simulink model "torqueWalkingR2012b"  (Simulink 8.0)
settings: Solver=FixedStepDiscrete  StartTime=0.0  StopTime=Config.t_end  FixedStep=Config.t_step  RelTol=1e-3
InitFcn:
  | cd(fileparts(which(bdroot)));
  | initTorqueWalking;
StopFcn:
  | disp_early_termination
undefined symbols (not defined in the file or in its folder): biasVectorConstraint_feet, Config, ConstraintMatrix_feet, DiscIntNeverNeededParam, Gains, ROBOT_DOF, Sat
libraries: WBToolboxLibrary x114, simulink x2
(part 2 of 4)

== system torqueWalkingR2012b/Robot State and References/State Machines ==
  Compute Feet to Base Link Transforms : Subsystem
  Compute State Velocity : Subsystem
  Constant6 : Constant  Value=eye(4)
  Get Estimate : WBToolboxLibrary/wholeBodyStates/Get Estimate  estimateType=Joints Position  robotName=WBT_robotName  localName=WBT_modelName  wbiFile=WBT_wbiFilename  wbiList=WBT_wbiList
  Get Estimate1 : WBToolboxLibrary/wholeBodyStates/Get Estimate  estimateType=Joints Velocity  robotName=WBT_robotName  localName=WBT_modelName  wbiFile=WBT_wbiFilename  wbiList=WBT_wbiList
  IMU measurements : WBToolboxLibrary/Utilities/Yarp Read  portName=Ports.IMU  signalSize=12  blocking=off  timestamp=off  autoconnect=on  errorOnConnection=off
  Select the Current State and References : Subsystem
  Selector1 : Selector  NumberOfDimensions=2  InputPortWidth=ROBOT_DOF  IndexOptions=Index vector (dialog),Index vector (dialog)  Indices=[1:ROBOT_DOF],1  OutputSizes=1,1
  s : Outport
  w_H_b : Outport  Port=2
  nu : Outport  Port=3
  feetInContact : Outport  Port=4
  state : Outport  Port=5
  references_LFoot : Outport  Port=6
  references_RFoot : Outport  Port=7
  references_CoM : Outport  Port=8
  references_rot_task : Outport  Port=9
  references_LHand : Outport  Port=10
  references_RHand : Outport  Port=11
  references_s : Outport  Port=12
  tag scope: feetInContact=global, nu=global, s=global, s_des=global, sd=global, state=global, w_H_b=global
  wires:
  Get Estimate/1 -> Compute State Velocity/2(s), s/1, [s], Select the Current State and References/1(s), Compute Feet to Base Link Transforms/1(s)
  Constant6/1 -> Compute Feet to Base Link Transforms/2(w_H_base_fixed)
  IMU measurements/1 -> Compute Feet to Base Link Transforms/3(IMU port)
  Compute Feet to Base Link Transforms/1(fixed_link_H_b) -> Select the Current State and References/2(fixed_link_H_b)
  Select the Current State and References/1(w_H_b) -> w_H_b/1, [w_H_b], Compute State Velocity/3(w_H_b)
  Select the Current State and References/2(feetInContact) -> feetInContact/1, [feetInContact], Compute State Velocity/4("feetInContact ")
  Compute State Velocity/1(nu) -> nu/1, [nu]
  Select the Current State and References/3(state) -> [state], state/1
  Select the Current State and References/10(references_s) -> references_s/1, Selector1/1
  Select the Current State and References/6(references_CoM) -> references_CoM/1
  Select the Current State and References/7(references_rot_task) -> references_rot_task/1
  Select the Current State and References/5(references_RFoot) -> references_RFoot/1
  Select the Current State and References/4(references_LFoot) -> references_LFoot/1
  Selector1/1 -> [s_des]
  Compute Feet to Base Link Transforms/2(LFoot_H_b) -> Select the Current State and References/3(LFoot_H_b)
  Compute Feet to Base Link Transforms/3(RFoot_H_b) -> Select the Current State and References/4(RFoot_H_b)
  Select the Current State and References/8(references_LHand) -> references_LHand/1
  Select the Current State and References/9(references_RHand) -> references_RHand/1
  Get Estimate1/1 -> [sd], Compute State Velocity/1(Joints velocity)

== system torqueWalkingR2012b/Subsystem/ZMP, support polygon ==
  f_Lfoot : Inport
  f_Rfoot : Inport  Port=2
  pose_lFoot : Inport  Port=3
  orient_lFoot : Inport  Port=4
  pose_rFoot : Inport  Port=5
  orient_rFoot : Inport  Port=6
  feetInContact : Inport  Port=7
  state : Inport  Port=8
  compute ZMP : MATLAB Function  TreatAsAtomicUnit=on
      settings: PermitHierarchicalResolution=ParametersOnly
  supportPolygon : MATLAB Function  TreatAsAtomicUnit=on
      settings: PermitHierarchicalResolution=ParametersOnly
  zmp : Outport
  support_polygon : Outport  Port=2
  tag scope: ZMP=global, support_polygon=global
  wires:
  pose_lFoot/1 -> supportPolygon/1(pose_lFoot), compute ZMP/3(pose_lFoot)
  pose_rFoot/1 -> compute ZMP/5(pose_rFoot), supportPolygon/2(pose_rFoot)
  compute ZMP/1(ZMP) -> zmp/1, [ZMP]
  f_Lfoot/1 -> compute ZMP/1(f_lFoot)
  f_Rfoot/1 -> compute ZMP/2(f_rFoot)
  orient_lFoot/1 -> compute ZMP/4(orient_lFoot)
  orient_rFoot/1 -> compute ZMP/6(orient_rFoot)
  feetInContact/1 -> compute ZMP/7(feetInContact), supportPolygon/3(feet_in_contact)
  supportPolygon/1(supportPolygon) -> [support_polygon], support_polygon/1
  state/1 -> supportPolygon/4(state)

== system torqueWalkingR2012b/Subsystem/task errors ==
  pos_vel_CoM : Inport
  pos_vel_acc_CoM_des : Inport  Port=2
  orient_vel_rot_rask : Inport  Port=3
  pos_vel_acc_rot_task_des : Inport  Port=4
  pose_vel_LFoot : Inport  Port=5
  pos_vel_acc_LFoot_des : Inport  Port=6
  pose_vel_RFoot : Inport  Port=7
  pos_vel_acc_RFoot_des : Inport  Port=8
  Rotation Error Left Foot : Subsystem
  Rotation Error Left Foot1 : Subsystem
  Rotation Error Rotational Task : Subsystem
  Selector{,2..6} (6 alike) : Selector  NumberOfDimensions=2  InputPortWidth=3  IndexOptions=Index vector (dialog),Index vector (dialog)  Indices=[1:3],1  OutputSizes=1,1
  Selector12 : Selector  NumberOfDimensions=2  InputPortWidth=3  IndexOptions=Index vector (dialog),Index vector (dialog)  Indices=[1:3],[1:3]  OutputSizes=1,1
  Selector13 : Selector  NumberOfDimensions=2  InputPortWidth=3  IndexOptions=Index vector (dialog),Index vector (dialog)  Indices=[1:3],[1:3]  OutputSizes=1,1
  Selector{7..9,15} (4 alike) : Selector  NumberOfDimensions=2  InputPortWidth=3  IndexOptions=Index vector (dialog),Index vector (dialog)  Indices=[4:6],[1:3]  OutputSizes=1,1
  Sum : Sum  Inputs=+-|
  Sum2 : Sum  Inputs=+-|
  Sum3 : Sum  Inputs=+-|
  Vector Concatenate : Concatenate  NumInputs=6
  taskErrors : Outport
  wires:
  Rotation Error Left Foot/1(|1-R^T*RDes|^2) -> Vector Concatenate/4
  Sum3/1 -> Vector Concatenate/5
  Sum2/1 -> Vector Concatenate/3
  Selector6/1 -> Sum3/2
  Selector5/1 -> Sum3/1
  pose_vel_LFoot/1 -> Selector3/1, Selector7/1
  pose_vel_RFoot/1 -> Selector9/1, Selector5/1
  Selector4/1 -> Sum2/2
  Selector/1 -> Sum/1
  Rotation Error Left Foot1/1(|1-R^T*RDes|^2) -> Vector Concatenate/6
  Selector13/1 -> Rotation Error Rotational Task/1(w_R_rot_task)
  Selector12/1 -> Rotation Error Rotational Task/2(w_R_rot_task_des)
  pos_vel_acc_LFoot_des/1 -> Selector15/1, Selector4/1
  Selector15/1 -> Rotation Error Left Foot/2(w_R_RFoot_des)
  Sum/1 -> Vector Concatenate/1
  Rotation Error Rotational Task/1(|1-R^T*RDes|^2) -> Vector Concatenate/2
  Selector8/1 -> Rotation Error Left Foot1/2(w_R_RFoot_des)
  orient_vel_rot_rask/1 -> Selector13/1
  Selector2/1 -> Sum/2
  Selector9/1 -> Rotation Error Left Foot1/1(w_R_RFoot)
  Selector3/1 -> Sum2/1
  pos_vel_acc_rot_task_des/1 -> Selector12/1
  pos_vel_acc_RFoot_des/1 -> Selector8/1, Selector6/1
  pos_vel_CoM/1 -> Selector/1
  Selector7/1 -> Rotation Error Left Foot/1(w_R_RFoot)
  pos_vel_acc_CoM_des/1 -> Selector2/1
  Vector Concatenate/1 -> taskErrors/1

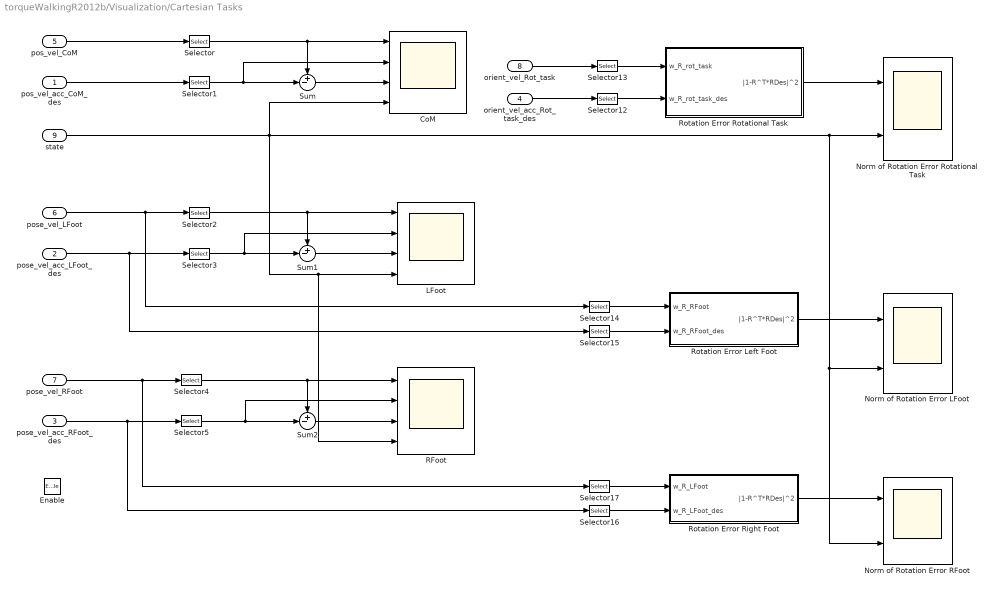
== system torqueWalkingR2012b/Visualization/Cartesian Tasks ==
  pos_vel_acc_CoM_des : Inport
  pose_vel_acc_LFoot_des : Inport  Port=2
  pose_vel_acc_RFoot_des : Inport  Port=3
  orient_vel_acc_Rot_task_des : Inport  Port=4
  pos_vel_CoM : Inport  Port=5
  pose_vel_LFoot : Inport  Port=6
  pose_vel_RFoot : Inport  Port=7
  orient_vel_Rot_task : Inport  Port=8
  state : Inport  Port=9
  Enable : EnablePort
  CoM : Scope  NumInputPorts=4
      settings: TimeRange=auto  ShowLegends=on  MaxDataPoints=5000  SaveName=forKin_CoM_DATA  YMin=-0.22134~-0.21729~-0.00986~0.5  YMax=0.60585~0.59423~0.01226~5.5  SampleTime=-1
  LFoot : Scope  NumInputPorts=4
      settings: TimeRange=auto  MaxDataPoints=5000  SaveName=forKin_LFoot_DATA  YMin=-0.0302~-0.02873~-0.00903~0.5  YMax=0.0249~0.02873~0.00291~5.5  SampleTime=-1
  Norm of Rotation Error LFoot : Scope  NumInputPorts=2
      settings: TimeRange=auto  MaxDataPoints=5000  SaveName=ScopeData2  YMin=-0.000002~0.5  YMax=0.000022~5.5  SampleTime=-1
  Norm of Rotation Error RFoot : Scope  NumInputPorts=2
      settings: TimeRange=auto  MaxDataPoints=5000  SaveName=ScopeData3  YMin=-0.00046~0.5  YMax=0.00415~5.5  SampleTime=-1
  Norm of Rotation Error Rotational Task : Scope  NumInputPorts=2
      settings: TimeRange=auto  MaxDataPoints=5000  YMin=-0.07412~0.9  YMax=0.66711~1.1  SampleTime=-1
  RFoot : Scope  NumInputPorts=4
      settings: TimeRange=auto  ShowLegends=on  MaxDataPoints=5000  SaveName=forKin_RFoot_DATA  YMin=-0.16101~-0.15882~-0.00115~0.5  YMax=0.03981~0.0433~0.00043~5.5  SampleTime=-1
  Rotation Error Left Foot : Subsystem
  Rotation Error Right Foot : Subsystem
  Rotation Error Rotational Task : Subsystem
  Selector{,1..5} (6 alike) : Selector  NumberOfDimensions=2  InputPortWidth=3  IndexOptions=Index vector (dialog),Index vector (dialog)  Indices=[1:3],1  OutputSizes=1,1
  Selector12 : Selector  NumberOfDimensions=2  InputPortWidth=3  IndexOptions=Index vector (dialog),Index vector (dialog)  Indices=[1:3],[1:3]  OutputSizes=1,1
  Selector13 : Selector  NumberOfDimensions=2  InputPortWidth=3  IndexOptions=Index vector (dialog),Index vector (dialog)  Indices=[1:3],[1:3]  OutputSizes=1,1
  Selector{14..17} (4 alike) : Selector  NumberOfDimensions=2  InputPortWidth=3  IndexOptions=Index vector (dialog),Index vector (dialog)  Indices=[4:6],[1:3]  OutputSizes=1,1
  Sum : Sum  Inputs=+-|
  Sum1 : Sum  Inputs=+-|
  Sum2 : Sum  Inputs=+-|
  wires:
  Selector1/1 -> CoM/2, Sum/2
  pos_vel_CoM/1 -> Selector/1
  pos_vel_acc_CoM_des/1 -> Selector1/1
  Selector2/1 -> Sum1/1, LFoot/1
  Selector3/1 -> Sum1/2, LFoot/2
  Selector4/1 -> Sum2/1, RFoot/1
  Selector5/1 -> RFoot/2, Sum2/2
  pose_vel_RFoot/1 -> Selector4/1, Selector17/1
  state/1 -> Norm of Rotation Error RFoot/2, Norm of Rotation Error LFoot/2, Norm of Rotation Error Rotational Task/2, CoM/4, RFoot/4, LFoot/4
  pose_vel_acc_RFoot_des/1 -> Selector5/1, Selector16/1
  pose_vel_LFoot/1 -> Selector2/1, Selector14/1
  Selector12/1 -> Rotation Error Rotational Task/2(w_R_rot_task_des)
  pose_vel_acc_LFoot_des/1 -> Selector15/1, Selector3/1
  orient_vel_acc_Rot_task_des/1 -> Selector12/1
  orient_vel_Rot_task/1 -> Selector13/1
  Selector/1 -> Sum/1, CoM/1
  Sum/1 -> CoM/3
  Sum1/1 -> LFoot/3
  Sum2/1 -> RFoot/3
  Rotation Error Rotational Task/1(|1-R^T*RDes|^2) -> Norm of Rotation Error Rotational Task/1
  Selector13/1 -> Rotation Error Rotational Task/1(w_R_rot_task)
  Rotation Error Left Foot/1(|1-R^T*RDes|^2) -> Norm of Rotation Error LFoot/1
  Selector14/1 -> Rotation Error Left Foot/1(w_R_RFoot)
  Selector15/1 -> Rotation Error Left Foot/2(w_R_RFoot_des)
  Rotation Error Right Foot/1(|1-R^T*RDes|^2) -> Norm of Rotation Error RFoot/1
  Selector16/1 -> Rotation Error Right Foot/2(w_R_LFoot_des)
  Selector17/1 -> Rotation Error Right Foot/1(w_R_LFoot)

== system torqueWalkingR2012b/Visualization/Emergency Stop ==
  note: Stop the simulation when the force on each feet is below a threshold (i.e. robot falls)
  F_l_foot : Inport
  F_r_foot : Inport  Port=2
  Enable : EnablePort
  Compare To Constant : simulink/Logic and Bit Operations/Compare To Constant  relop=<=  const=50  OutDataTypeStr=boolean
  Compare To Constant1 : simulink/Logic and Bit Operations/Compare To Constant  relop=<=  const=50  OutDataTypeStr=boolean
  Constant3 : Constant  Value=0  OutDataTypeStr=boolean
  Constant4 : Constant  OutDataTypeStr=boolean
  Logical Operator : Logic  AllPortsSameDT=off  OutDataTypeStr=boolean
  Stop Simulation : Stop
  Switch1 : Switch  Criteria=u2 ~= 0  Threshold=0.5
  To Workspace : ToWorkspace  VariableName=no_force_on_feet  SaveFormat=Timeseries  SampleTime=-1
      settings: MaxDataPoints=1
  select_pose5 : Selector  InputPortWidth=6  IndexOptions=Index vector (dialog)  Indices=[3]  OutputSizes=1
  select_pose6 : Selector  InputPortWidth=6  IndexOptions=Index vector (dialog)  Indices=[3]  OutputSizes=1
  wires:
  F_l_foot/1 -> select_pose5/1
  F_r_foot/1 -> select_pose6/1
  Compare To Constant/1 -> Logical Operator/1
  Compare To Constant1/1 -> Logical Operator/2
  Logical Operator/1 -> Switch1/2
  Switch1/1 -> To Workspace/1, Stop Simulation/1
  Constant4/1 -> Switch1/1
  Constant3/1 -> Switch1/3
  select_pose5/1 -> Compare To Constant/1
  select_pose6/1 -> Compare To Constant1/1

== system torqueWalkingR2012b/Visualization/Emergency Stop1 ==
  exitFlagQP : Inport
  Enable : EnablePort
  Constant : Constant  Value=2
  Constant1 : Constant  Value=0  OutDataTypeStr=boolean
  Constant2 : Constant  OutDataTypeStr=boolean
  Stop Simulation : Stop
  Sum : Sum  Inputs=|++
  Switch : Switch  Criteria=u2 > Threshold  Threshold=0.1
  To Workspace : ToWorkspace  VariableName=exitFlagQP_unsuccessful  SaveFormat=Timeseries  SampleTime=-1
      settings: MaxDataPoints=1
  wires:
  exitFlagQP/1 -> Sum/1
  Sum/1 -> Switch/2
  Constant/1 -> Sum/2
  Constant1/1 -> Switch/1
  Constant2/1 -> Switch/3
  Switch/1 -> To Workspace/1, Stop Simulation/1

== system torqueWalkingR2012b/Visualization/Emergency Stop2 ==
  note: Stop the simulation when the ZMP goes out of the support polygon
  ZMP : Inport
  support_polygon : Inport  Port=2
  Enable : EnablePort
  Constant3 : Constant  Value=0  OutDataTypeStr=boolean
  Constant4 : Constant  OutDataTypeStr=boolean
  Logical Operator : Logic  Operator=OR  AllPortsSameDT=off  OutDataTypeStr=boolean
  Relational Operator : RelationalOperator  Operator=<  OutDataTypeStr=boolean
  Relational Operator1 : RelationalOperator  Operator=>  OutDataTypeStr=boolean
  Stop Simulation : Stop
  Sum of Elements : Sum  Inputs=+
  Switch1 : Switch  Criteria=u2 ~= 0  Threshold=0.5
  To Workspace : ToWorkspace  VariableName=ZMP_out_of_bounds  SaveFormat=Timeseries  SampleTime=-1
      settings: MaxDataPoints=1
  select_pose1 : Selector  NumberOfDimensions=2  InputPortWidth=6  IndexOptions=Index vector (dialog),Index vector (dialog)  Indices=[1 2],2  OutputSizes=1,1
  select_pose6 : Selector  NumberOfDimensions=2  InputPortWidth=6  IndexOptions=Index vector (dialog),Index vector (dialog)  Indices=[1 2],1  OutputSizes=1,1
  wires:
  Constant3/1 -> Switch1/3
  Constant4/1 -> Switch1/1
  Switch1/1 -> To Workspace/1, Stop Simulation/1
  Sum of Elements/1 -> Switch1/2
  ZMP/1 -> Relational Operator1/1, Relational Operator/1
  select_pose6/1 -> Relational Operator/2
  select_pose1/1 -> Relational Operator1/2
  Relational Operator/1 -> Logical Operator/1
  Relational Operator1/1 -> Logical Operator/2
  Logical Operator/1 -> Sum of Elements/1
  support_polygon/1 -> select_pose1/1, select_pose6/1

== system torqueWalkingR2012b/Visualization/Forces and Torques ==
  tau measured : Inport
  tau desired : Inport  Port=2
  f LFoot desired : Inport  Port=3
  f RFoot desired : Inport  Port=4
  exitFlag QP : Inport  Port=5
  f LFoot : Inport  Port=6
  f RFoot : Inport  Port=7
  state : Inport  Port=8
  Enable : EnablePort
  Demux{1..4} (4 alike) : Demux  Outputs=[3;3]
  DoFs converter : WBToolboxLibrary/Utilities/DoFs converter  yarp2WBIOption=From WBI to YARP  robotName=WBT_robotName  localName=WBT_modelName  wbiFile=WBT_wbiFilename  wbiList=WBT_wbiList
  DoFs converter1 : WBToolboxLibrary/Utilities/DoFs converter  yarp2WBIOption=From WBI to YARP  robotName=WBT_robotName  localName=WBT_modelName  wbiFile=WBT_wbiFilename  wbiList=WBT_wbiList
  DoFs converter2 : WBToolboxLibrary/Utilities/DoFs converter  yarp2WBIOption=From WBI to YARP  robotName=WBT_robotName  localName=WBT_modelName  wbiFile=WBT_wbiFilename  wbiList=WBT_wbiList
  QP status : Scope  NumInputPorts=2
      settings: TimeRange=auto  MaxDataPoints=5000  SaveName=exitFlagQP_DATA  YMin=-1.00000~0.5  YMax=1.00000~5.5  SampleTime=-1
  Sum : Sum  Inputs=+-|
  Sum1 : Sum  Inputs=|+-
  Sum2 : Sum  Inputs=+-|
  Sum3 : Sum  Inputs=|+-
  Sum4 : Sum  Inputs=+-|
  desired torque : Scope  NumInputPorts=6
      settings: TimeRange=14  ShowLegends=on  MaxDataPoints=5000  SaveName=tauDes_DATA  YMin=-13.18648~-6.43141~-7.08568~-19.20891~-19.28381~0.9  YMax=1.62552~17.66798~17.45574~30.97955~31.09849~1.1  SampleTime=-1
  forces Left Foot : Scope  NumInputPorts=4
      settings: TimeRange=40  ShowLegends=on  MaxDataPoints=5000  SaveName=LFoot_forces_DATA  YMin=-49.37639~-39.54867~-105.83056~0.5  YMax=334.90823~335.47986~63.27597~5.5  SampleTime=-1
  forces Right Foot : Scope  NumInputPorts=4
      settings: TimeRange=40  MaxDataPoints=5000  SaveName=RFoot_forces_DATA  YMin=-91.98017~-26.56964~-91.98017~0.5  YMax=330.78868~185.22903~330.78868~5.5  SampleTime=-1
  measured torque : Scope  NumInputPorts=6
      settings: TimeRange=14  ShowLegends=on  MaxDataPoints=5000  SaveName=tauMeas_DATA  YMin=-5.91681~-2.23213~-2.22376~-3.66223~-3.58411~0.9  YMax=0.65763~1.82348~1.82041~3.39258~3.91053~1.1  SampleTime=-1
  moments Left Foot : Scope  NumInputPorts=4
      settings: TimeRange=40  MaxDataPoints=5000  SaveName=LFoot_moments_DATA  YMin=-7.05587~-8.99127~-14.1598~0.5  YMax=8.48162~7.11363~17.47181~5.5  SampleTime=-1
  moments Right Foot : Scope  NumInputPorts=4
      settings: TimeRange=40  MaxDataPoints=5000  SaveName=RFoot_moments_DATA  YMin=-3.70848~-4.31254~-7.21108~0.625  YMax=4.52341~3.56092~8.80515~4.375  SampleTime=-1
  torque error : Scope  NumInputPorts=6
      settings: TimeRange=14  ShowLegends=on  MaxDataPoints=5000  SaveName=tauErr_DATA  YMin=-21.19301~-15.40032~-16.23554~-28.77317~-27.38859~0.75  YMax=25.49644~20.6188~19.45962~25.35579~25.11667~3.25  SampleTime=-1
  wires:
  Sum2/1 -> moments Left Foot/3  "moments measured left foot"
  state/1 -> QP status/2, torque error/6, desired torque/6, forces Right Foot/4, moments Right Foot/4, forces Left Foot/4, moments Left Foot/4, measured torque/6
  DoFs converter1/2 -> desired torque/2  "left_arm"
  Demux4/1 -> forces Left Foot/2, Sum1/2  "force desired left foot"
  DoFs converter2/1 -> torque error/1  "torso"
  DoFs converter1/4 -> desired torque/4  "left_leg"
  Demux4/2 -> moments Left Foot/2, Sum2/2  "moments measured left foot"
  DoFs converter/1 -> measured torque/1  "torso"
  DoFs converter2/3 -> torque error/3  "right_arm"
  f RFoot desired/1 -> Demux3/1
  DoFs converter1/1 -> desired torque/1  "torso"
  Sum4/1 -> moments Right Foot/3  "moments measured right foot"
  tau desired/1 -> Sum/2, DoFs converter1/1
  Demux2/1 -> forces Right Foot/1, Sum3/1  "force measured right foot"
  DoFs converter2/2 -> torque error/2  "left_arm"
  Sum3/1 -> forces Right Foot/3  "force error right foot"
  DoFs converter/5 -> measured torque/5  "right_leg"
  DoFs converter2/5 -> torque error/5  "right_leg"
  exitFlag QP/1 -> QP status/1
  f LFoot/1 -> Demux1/1  "wL_WBDT"
  DoFs converter1/3 -> desired torque/3  "right_arm"
  Demux3/1 -> forces Right Foot/2, Sum3/2  "force desired right foot"
  f LFoot desired/1 -> Demux4/1
  Sum1/1 -> forces Left Foot/3  "force error left foot"
  tau measured/1 -> Sum/1, DoFs converter/1
  DoFs converter1/5 -> desired torque/5  "right_leg"
  DoFs converter/2 -> measured torque/2  "left_arm"
  DoFs converter/3 -> measured torque/3  "right_arm"
  Demux3/2 -> moments Right Foot/2, Sum4/2  "moments measured right foot"
  Sum/1 -> DoFs converter2/1
  Demux1/1 -> forces Left Foot/1, Sum1/1  "force measured left foot"
  DoFs converter/4 -> measured torque/4  "left_leg"
  Demux1/2 -> moments Left Foot/1, Sum2/1  "moments measured left foot"
  f RFoot/1 -> Demux2/1  "wR_WBDT"
  DoFs converter2/4 -> torque error/4  "left_leg"
  Demux2/2 -> moments Right Foot/1, Sum4/1  "moments measured right foot"

== system torqueWalkingR2012b/Visualization/Gain Scheduling ==
  Kp_CoM : Inport
  Kd_CoM : Inport  Port=2
  Kp_LFoot : Inport  Port=3
  Kd_LFoot : Inport  Port=4
  Kp_RFoot : Inport  Port=5
  Kd_RFoot : Inport  Port=6
  Kp_rot_task : Inport  Port=7
  Kd_rot_task : Inport  Port=8
  impedances : Inport  Port=9
  dampings : Inport  Port=10
  state : Inport  Port=11
  Enable : EnablePort
  DoFs converter1 : WBToolboxLibrary/Utilities/DoFs converter  yarp2WBIOption=From WBI to YARP  robotName=WBT_robotName  localName=WBT_modelName  wbiFile=WBT_wbiFilename  wbiList=WBT_wbiList
  DoFs converter4 : WBToolboxLibrary/Utilities/DoFs converter  yarp2WBIOption=From WBI to YARP  robotName=WBT_robotName  localName=WBT_modelName  wbiFile=WBT_wbiFilename  wbiList=WBT_wbiList
  joint position gains : Scope  NumInputPorts=6
      settings: TimeRange=auto  MaxDataPoints=5000  SaveName=impedances_DATA  YMin=-10~-10~-10~-10~-10~-10  YMax=10~10~10~10~10~10  SampleTime=-1
  joint valocity gains : Scope  NumInputPorts=6
      settings: TimeRange=auto  MaxDataPoints=5000  SaveName=dampings_DATA  YMin=-10~-10~-10~-10~-10~-10  YMax=10~10~10~10~10~10  SampleTime=-1
  orient gains rot task : Scope  NumInputPorts=2
      settings: TimeRange=auto  MaxDataPoints=5000  SaveName=Kp_rot_task_DATA  YMin=-0.15075~0.9  YMax=0.68063~1.1  SampleTime=-1
  pos gains CoM : Scope  NumInputPorts=2
      settings: TimeRange=auto  MaxDataPoints=5000  SaveName=Kp_CoM_DATA  YMin=40.00000~0.75  YMax=60.00000~3.25  SampleTime=-1
  pose gains LFoot : Scope  NumInputPorts=2
      settings: TimeRange=auto  MaxDataPoints=5000  SaveName=Kp_LFoot_DATA  YMin=27.5~0.75  YMax=52.5~3.25  SampleTime=-1
  pose gains RFoot : Scope  NumInputPorts=2
      settings: TimeRange=auto  MaxDataPoints=5000  SaveName=Kp_RFoot_DATA  YMin=-0.15075~0.9  YMax=0.68063~1.1  SampleTime=-1
  vel gains CoM : Scope  NumInputPorts=2
      settings: TimeRange=auto  MaxDataPoints=5000  SaveName=Kd_CoM_DATA  YMin=12.3762~0.625  YMax=15.10531~4.375  SampleTime=-1
  vel gains LFoot : Scope  NumInputPorts=2
      settings: TimeRange=auto  MaxDataPoints=5000  SaveName=Kd_LFoot_DATA  YMin=10.55599~0.75  YMax=14.5406~3.25  SampleTime=-1
  vel gains RFoot : Scope  NumInputPorts=2
      settings: TimeRange=auto  MaxDataPoints=5000  SaveName=Kd_RFoot_DATA  YMin=-0.15075~0.9  YMax=0.68063~1.1  SampleTime=-1
  vel gains rot task : Scope  NumInputPorts=2
      settings: TimeRange=auto  MaxDataPoints=5000  SaveName=Kd_rot_task_DATA  YMin=-0.15075~0.9  YMax=0.68063~1.1  SampleTime=-1
  wires:
  Kp_CoM/1 -> pos gains CoM/1
  Kp_LFoot/1 -> pose gains LFoot/1
  Kp_RFoot/1 -> pose gains RFoot/1
  Kp_rot_task/1 -> orient gains rot task/1
  state/1 -> vel gains LFoot/2, pose gains LFoot/2, vel gains CoM/2, vel gains rot task/2, orient gains rot task/2, vel gains RFoot/2, joint valocity gains/6, joint position gains/6, pose gains RFoot/2, pos gains CoM/2
  Kd_CoM/1 -> vel gains CoM/1
  Kd_LFoot/1 -> vel gains LFoot/1
  Kd_RFoot/1 -> vel gains RFoot/1
  Kd_rot_task/1 -> vel gains rot task/1
  DoFs converter4/2 -> joint position gains/2  "left_arm"
  DoFs converter4/1 -> joint position gains/1  "torso"
  DoFs converter4/4 -> joint position gains/4  "left_leg"
  DoFs converter4/3 -> joint position gains/3  "right_arm"
  DoFs converter4/5 -> joint position gains/5  "right_leg"
  DoFs converter1/2 -> joint valocity gains/2  "left_arm"
  DoFs converter1/1 -> joint valocity gains/1  "torso"
  DoFs converter1/4 -> joint valocity gains/4  "left_leg"
  DoFs converter1/3 -> joint valocity gains/3  "right_arm"
  DoFs converter1/5 -> joint valocity gains/5  "right_leg"
  impedances/1 -> DoFs converter4/1
  dampings/1 -> DoFs converter1/1

== system torqueWalkingR2012b/Visualization/Joints and Floating Base State ==
  s : Inport
  w_H_b : Inport  Port=2
  nu : Inport  Port=3
  state : Inport  Port=4
  s_des : Inport  Port=5
  feetInContact : Inport  Port=6
  Enable : EnablePort
  DoFs converter{,1..3} (4 alike) : WBToolboxLibrary/Utilities/DoFs converter  yarp2WBIOption=From WBI to YARP  robotName=WBT_robotName  localName=WBT_modelName  wbiFile=WBT_wbiFilename  wbiList=WBT_wbiList
  Gain : Gain  Gain=180/pi
  Gain1 : Gain  Gain=180/pi
  Gain2 : Gain  Gain=180/pi
  Selector : Selector  NumberOfDimensions=2  InputPortWidth=3  IndexOptions=Index vector (dialog),Index vector (dialog)  Indices=[1:3],4  OutputSizes=1,1
  Selector1 : Selector  InputPortWidth=ROBOT_DOF+6  IndexOptions=Index vector (dialog)  Indices=[1:6]  OutputSizes=1
  Selector2 : Selector  InputPortWidth=ROBOT_DOF+6  IndexOptions=Index vector (dialog)  Indices=[7:ROBOT_DOF+6]  OutputSizes=1
  Sum : Sum  Inputs=+-|
  base position : Scope  NumInputPorts=2
      settings: TimeRange=auto  MaxDataPoints=5000  SaveName=basePos_DATA  YMin=-0.20029~0.75  YMax=0.92593~3.25  SampleTime=-1
  base velocity : Scope  NumInputPorts=2
      settings: TimeRange=auto  MaxDataPoints=5000  SaveName=baseVel_DATA  YMin=-0.41349~0.75  YMax=0.49364~3.25  SampleTime=-1
  desired joint pos : Scope  NumInputPorts=6
      settings: TimeRange=auto  MaxDataPoints=5000  SaveName=jointDes_DATA  YMin=-1.73238~-39.09396~-39.16347~-0.13035~-0.1588~0.9  YMax=-0.13168~54.24597~54.26229~0.09217~0.03558~1.1  SampleTime=-1
  feet in contact : Scope  NumInputPorts=2
      settings: TimeRange=auto  MaxDataPoints=5000  SaveName=feetInContact_DATA  YMin=-0.125~0.5  YMax=1.125~5.5  SampleTime=-1
  joint error : Scope  NumInputPorts=6
      settings: TimeRange=auto  MaxDataPoints=5000  SaveName=jointErr_DATA  YMin=-10.0481~-14.25395~-12.82312~-15.16191~-15.05108~0.75  YMax=10.63111~10.66532~10.34559~9.36985~9.54972~3.25  SampleTime=-1
  joint velocity : Scope  NumInputPorts=6
      settings: TimeRange=auto  MaxDataPoints=5000  SaveName=jointVel_DATA  YMin=-22.02483~-54.17338~-59.81389~-28.54859~-29.79467~0.75  YMax=21.72199~42.41291~49.23324~62.06883~60.67695~3.25  SampleTime=-1
  measured joint pos : Scope  NumInputPorts=6
      settings: TimeRange=auto  MaxDataPoints=5000  SaveName=jointMeas_DATA  YMin=-12.2455~-64.79663~-127.11597~-45.09359~-43.9411~0.75  YMax=70.11382~60.78722~193.40456~24.67766~34.7354~3.25  SampleTime=-1
  wires:
  DoFs converter1/2 -> desired joint pos/2  "left_arm"
  DoFs converter/5 -> measured joint pos/5  "right_leg"
  DoFs converter2/1 -> joint error/1  "torso"
  DoFs converter/4 -> measured joint pos/4  "left_leg"
  DoFs converter/2 -> measured joint pos/2  "left_arm"
  s/1 -> Gain/1
  DoFs converter1/1 -> desired joint pos/1  "torso"
  DoFs converter1/4 -> desired joint pos/4  "left_leg"
  DoFs converter1/3 -> desired joint pos/3  "right_arm"
  DoFs converter/3 -> measured joint pos/3  "right_arm"
  DoFs converter2/5 -> joint error/5  "right_leg"
  DoFs converter2/2 -> joint error/2  "left_arm"
  DoFs converter/1 -> measured joint pos/1  "torso"
  s_des/1 -> Gain1/1
  DoFs converter1/5 -> desired joint pos/5  "right_leg"
  DoFs converter2/4 -> joint error/4  "left_leg"
  DoFs converter2/3 -> joint error/3  "right_arm"
  DoFs converter3/5 -> joint velocity/5  "right_leg"
  DoFs converter3/1 -> joint velocity/1  "torso"
  DoFs converter3/4 -> joint velocity/4  "left_leg"
  DoFs converter3/3 -> joint velocity/3  "right_arm"
  DoFs converter3/2 -> joint velocity/2  "left_arm"
  nu/1 -> Selector2/1, Selector1/1
  w_H_b/1 -> Selector/1
  Gain/1 -> Sum/1, DoFs converter/1
  Gain1/1 -> Sum/2, DoFs converter1/1
  Gain2/1 -> DoFs converter3/1
  Selector/1 -> base position/1
  Selector2/1 -> Gain2/1
  state/1 -> measured joint pos/6, joint velocity/6, base velocity/2, feet in contact/2, base position/2, joint error/6, desired joint pos/6
  Selector1/1 -> base velocity/1
  feetInContact/1 -> feet in contact/1
  Sum/1 -> DoFs converter2/1

== system torqueWalkingR2012b/Visualization/Orientation Tasks References ==
  w_R_LFoot_des : Inport
  w_R_RFoot_des : Inport  Port=2
  w_R_rot_task_des : Inport  Port=3
  w_R_LFoot : Inport  Port=4
  w_R_RFoot : Inport  Port=5
  w_R_rot_task : Inport  Port=6
  omegaDot_LFoot : Inport  Port=7
  omegaDot_RFoot : Inport  Port=8
  omegaDot_rot_task : Inport  Port=9
  omega_rot_task : Inport  Port=10
  omega_RFoot : Inport  Port=11
  omega_LFoot : Inport  Port=12
  Enable : EnablePort
  LFoot omega : Scope
      settings: TimeRange=auto  MaxDataPoints=5000  SaveName=omega_LFoot_DATA  YMin=-0.0000000000000000000076  YMax=0.0000000000000000000008  SampleTime=-1
  LFoot omegaDot : Scope
      settings: TimeRange=auto  MaxDataPoints=5000  SaveName=omegaDot_LFoot_DATA  YMin=-0.000000000000000000034  YMax=0.00000000000000000003  SampleTime=-1
  Norm of Rotation Error LFoot : Scope
      settings: TimeRange=auto  MaxDataPoints=5000  SaveName=rotErr_LFoot_ref_DATA  YMin=0.000000000000000000000000000000197218  YMax=0.000000000000000000000000000000197236  SampleTime=-1
  Norm of Rotation Error RFoot : Scope
      settings: TimeRange=auto  MaxDataPoints=5000  SaveName=rotError_RFoot_ref_DATA  YMin=0.0000000000000000000000000000002108  YMax=0.0000000000000000000000000000002177  SampleTime=-1
  Norm of Rotation Error rot_task : Scope
      settings: TimeRange=auto  MaxDataPoints=5000  SaveName=rotErr_Root_ref_DATA  YMin=0.00000000000000000000000000000011  YMax=0.00000000000000000000000000000031  SampleTime=-1
  RFoot omega : Scope
      settings: TimeRange=auto  MaxDataPoints=5000  SaveName=omega_RFoot_DATA  YMin=-0.000000000000000000044  YMax=0.000000000000000000005  SampleTime=-1
  RFoot omegaDot : Scope
      settings: TimeRange=auto  MaxDataPoints=5000  SaveName=omegaDot_RFoot_DATA  YMin=-1.00000  YMax=1.00000  SampleTime=-1
  Rotation Error Left Foot : Subsystem
  Rotation Error Right Foot : Subsystem
  Rotation Error Rotational Task : Subsystem
  rot_task omega : Scope
      settings: TimeRange=auto  MaxDataPoints=5000  SaveName=omega_Root_DATA  YMin=-0.00478  YMax=0.008  SampleTime=-1
  rot_task omegaDot : Scope
      settings: TimeRange=auto  MaxDataPoints=5000  SaveName=omegaDot_Root_DATA  YMin=-0.00000000000000000000000000000000018  YMax=0.00000000000000000000000000000000023  SampleTime=-1
  wires:
  omega_rot_task/1 -> rot_task omega/1
  omega_RFoot/1 -> RFoot omega/1
  omega_LFoot/1 -> LFoot omega/1
  omegaDot_LFoot/1 -> LFoot omegaDot/1
  omegaDot_RFoot/1 -> RFoot omegaDot/1
  omegaDot_rot_task/1 -> rot_task omegaDot/1
  Rotation Error Left Foot/1(|1-R^T*RDes|^2) -> Norm of Rotation Error LFoot/1
  w_R_LFoot/1 -> Rotation Error Left Foot/1(w_R_LFoot)
  w_R_LFoot_des/1 -> Rotation Error Left Foot/2(w_R_LFoot_des)
  Rotation Error Right Foot/1(|1-R^T*RDes|^2) -> Norm of Rotation Error RFoot/1
  w_R_RFoot/1 -> Rotation Error Right Foot/1(w_R_RFoot)
  w_R_RFoot_des/1 -> Rotation Error Right Foot/2(w_R_RFoot_des)
  Rotation Error Rotational Task/1(|1-R^T*RDes|^2) -> Norm of Rotation Error rot_task/1
  w_R_rot_task/1 -> Rotation Error Rotational Task/1(w_R_rot_task)
  w_R_rot_task_des/1 -> Rotation Error Rotational Task/2(w_R_rot_task_des)

== system torqueWalkingR2012b/synchronizer/GAZEBO_SYNCHRONIZER ==
  Enable : EnablePort
  Simulator Synchronizer : WBToolboxLibrary/Utilities/Simulator Synchronizer  period=Config.t_step  serverPortName='/clock/rpc'  clientPortName='/WBT_synchronizer/rpc:o'

== system torqueWalkingR2012b/synchronizer/REAL_TIME_SYNC ==
  Enable : EnablePort
  Real Time Synchronizer : WBToolboxLibrary/Utilities/Real Time Synchronizer  period=Config.t_step

== system torqueWalkingR2012b/Dynamics and Kinematics/Compute Dynamic and Kinematic Quantities/Jacobians and JDot_nu ==
  s : Inport
  nu_b : Inport  Port=2
  sDot : Inport  Port=3
  w_H_b : Inport  Port=4
  DotJ Nu CoM : WBToolboxLibrary/wholeBodyModel/Jacobians/DotJ Nu  frameName=Frames.COM  robotName=WBT_robotName  localName=WBT_modelName  wbiFile=WBT_wbiFilename  wbiList=WBT_wbiList
  DotJ Nu LFoot : WBToolboxLibrary/wholeBodyModel/Jacobians/DotJ Nu  frameName=Frames.LEFT_FOOT  robotName=WBT_robotName  localName=WBT_modelName  wbiFile=WBT_wbiFilename  wbiList=WBT_wbiList
  DotJ Nu LHand : WBToolboxLibrary/wholeBodyModel/Jacobians/DotJ Nu  frameName=Frames.LEFT_HAND  robotName=WBT_robotName  localName=WBT_modelName  wbiFile=WBT_wbiFilename  wbiList=WBT_wbiList
  DotJ Nu RFoot : WBToolboxLibrary/wholeBodyModel/Jacobians/DotJ Nu  frameName=Frames.RIGHT_FOOT  robotName=WBT_robotName  localName=WBT_modelName  wbiFile=WBT_wbiFilename  wbiList=WBT_wbiList
  DotJ Nu RHand : WBToolboxLibrary/wholeBodyModel/Jacobians/DotJ Nu  frameName=Frames.RIGHT_HAND  robotName=WBT_robotName  localName=WBT_modelName  wbiFile=WBT_wbiFilename  wbiList=WBT_wbiList
  DotJ Nu rotational task : WBToolboxLibrary/wholeBodyModel/Jacobians/DotJ Nu  frameName=Frames.ROT_TASK_LINK  robotName=WBT_robotName  localName=WBT_modelName  wbiFile=WBT_wbiFilename  wbiList=WBT_wbiList
  Jacobian CoM : WBToolboxLibrary/wholeBodyModel/Jacobians/Jacobian  frameName=Frames.COM  robotName=WBT_robotName  localName=WBT_modelName  wbiFile=WBT_wbiFilename  wbiList=WBT_wbiList
  Jacobian LFoot : WBToolboxLibrary/wholeBodyModel/Jacobians/Jacobian  frameName=Frames.LEFT_FOOT  robotName=WBT_robotName  localName=WBT_modelName  wbiFile=WBT_wbiFilename  wbiList=WBT_wbiList
  Jacobian LHand : WBToolboxLibrary/wholeBodyModel/Jacobians/Jacobian  frameName=Frames.LEFT_HAND  robotName=WBT_robotName  localName=WBT_modelName  wbiFile=WBT_wbiFilename  wbiList=WBT_wbiList
  Jacobian RFoot : WBToolboxLibrary/wholeBodyModel/Jacobians/Jacobian  frameName=Frames.RIGHT_FOOT  robotName=WBT_robotName  localName=WBT_modelName  wbiFile=WBT_wbiFilename  wbiList=WBT_wbiList
  Jacobian RHand : WBToolboxLibrary/wholeBodyModel/Jacobians/Jacobian  frameName=Frames.RIGHT_HAND  robotName=WBT_robotName  localName=WBT_modelName  wbiFile=WBT_wbiFilename  wbiList=WBT_wbiList
  Jacobian rotational task : WBToolboxLibrary/wholeBodyModel/Jacobians/Jacobian  frameName=Frames.ROT_TASK_LINK  robotName=WBT_robotName  localName=WBT_modelName  wbiFile=WBT_wbiFilename  wbiList=WBT_wbiList
  J_LFoot : Outport
  J_RFoot : Outport  Port=2
  J_CoM : Outport  Port=3
  J_rot_task : Outport  Port=4
  J_LHand : Outport  Port=5
  J_RHand : Outport  Port=6
  JDot_nu_LFoot : Outport  Port=7
  JDot_nu_RFoot : Outport  Port=8
  JDot_nu_CoM : Outport  Port=9
  JDot_nu_rot_task : Outport  Port=10
  JDot_nu_LHand : Outport  Port=11
  JDot_nu_RHand : Outport  Port=12
  wires:
  Jacobian CoM/1 -> J_CoM/1
  Jacobian rotational task/1 -> J_rot_task/1
  Jacobian LFoot/1 -> J_LFoot/1
  Jacobian RFoot/1 -> J_RFoot/1
  w_H_b/1 -> Jacobian RHand/1, Jacobian LHand/1, Jacobian RFoot/1, Jacobian LFoot/1, DotJ Nu RHand/1, DotJ Nu LHand/1, DotJ Nu RFoot/1, DotJ Nu LFoot/1, DotJ Nu rotational task/1, DotJ Nu CoM/1, Jacobian CoM/1, Jacobian rotational task/1
  sDot/1 -> DotJ Nu RFoot/4, DotJ Nu RHand/4, DotJ Nu LHand/4, DotJ Nu LFoot/4, DotJ Nu rotational task/4, DotJ Nu CoM/4
  nu_b/1 -> DotJ Nu CoM/3, DotJ Nu RHand/3, DotJ Nu LHand/3, DotJ Nu RFoot/3, DotJ Nu LFoot/3, DotJ Nu rotational task/3
  s/1 -> Jacobian RHand/2, Jacobian LHand/2, DotJ Nu RHand/2, DotJ Nu LHand/2, DotJ Nu RFoot/2, DotJ Nu LFoot/2, DotJ Nu rotational task/2, DotJ Nu CoM/2, Jacobian RFoot/2, Jacobian CoM/2, Jacobian rotational task/2, Jacobian LFoot/2
  DotJ Nu RFoot/1 -> JDot_nu_RFoot/1
  DotJ Nu LFoot/1 -> JDot_nu_LFoot/1
  DotJ Nu rotational task/1 -> JDot_nu_rot_task/1
  DotJ Nu CoM/1 -> JDot_nu_CoM/1
  Jacobian RHand/1 -> J_RHand/1
  Jacobian LHand/1 -> J_LHand/1
  DotJ Nu LHand/1 -> JDot_nu_LHand/1
  DotJ Nu RHand/1 -> JDot_nu_RHand/1

== system torqueWalkingR2012b/Dynamics and Kinematics/Compute Dynamic and Kinematic Quantities/Mass Matrix and Bias Forces ==
  s : Inport
  nu_b : Inport  Port=2
  sDot : Inport  Port=3
  w_H_b : Inport  Port=4
  Add motors reflected inertias : Subsystem
  Get Bias Forces : WBToolboxLibrary/wholeBodyModel/Dynamics/Get Bias Forces  robotName=WBT_robotName  localName=WBT_modelName  wbiFile=WBT_wbiFilename  wbiList=WBT_wbiList  explicitGravity=off
  Mass Matrix : WBToolboxLibrary/wholeBodyModel/Dynamics/Mass Matrix  robotName=WBT_robotName  localName=WBT_modelName  wbiFile=WBT_wbiFilename  wbiList=WBT_wbiList
  h(q,nu) : Outport
  M(q) : Outport  Port=2
  wires:
  w_H_b/1 -> Mass Matrix/1, Get Bias Forces/1
  s/1 -> Mass Matrix/2, Get Bias Forces/2
  sDot/1 -> Get Bias Forces/4
  nu_b/1 -> Get Bias Forces/3
  Get Bias Forces/1 -> h(q,nu)/1
  Mass Matrix/1 -> Add motors reflected inertias/1(M)
  Add motors reflected inertias/1(M_with_motor_inertia) -> M(q)/1

== system torqueWalkingR2012b/Dynamics and Kinematics/Initial Conditions/Compute world to base transform ==
  s : Inport
  Constant : Constant  Value=Config.LFoot_in_contact_at0
  Constant6 : Constant  Value=eye(4)
  "Inv\\*  " : Product  Inputs=/*  Multiplication=Matrix(*)
  Switch6 : Switch  Criteria=u2 > Threshold
  left foot : WBToolboxLibrary/wholeBodyModel/Kinematics/Forward Kinematics  frameName=Frames.LEFT_FOOT  robotName=WBT_robotName  localName=WBT_modelName  wbiFile=WBT_wbiFilename  wbiList=WBT_wbiList
  left foot1 : WBToolboxLibrary/wholeBodyModel/Kinematics/Forward Kinematics  frameName=Frames.RIGHT_FOOT  robotName=WBT_robotName  localName=WBT_modelName  wbiFile=WBT_wbiFilename  wbiList=WBT_wbiList
  root_link : WBToolboxLibrary/wholeBodyModel/Kinematics/Forward Kinematics  frameName='root_link'  robotName=WBT_robotName  localName=WBT_modelName  wbiFile=WBT_wbiFilename  wbiList=WBT_wbiList
  w_H_b : Outport
  wires:
  Constant/1 -> Switch6/2
  left foot1/1 -> Switch6/1
  s/1 -> root_link/2, left foot/2, left foot1/2
  left foot/1 -> Switch6/3
  "Inv\\*  "/1 -> w_H_b/1
  Constant6/1 -> left foot/1, root_link/1, left foot1/1
  Switch6/1 -> "Inv\\*  "/1
  root_link/1 -> "Inv\\*  "/2

== system torqueWalkingR2012b/Dynamics and Kinematics/Initial Conditions/compute state velocity ==
  s : Inport
  w_H_b : Inport  Port=2
  "feetInContact " : Inport  Port=3
  sDot : Inport  Port=4
  Compute Base Velocity : MATLAB Function  TreatAsAtomicUnit=on
      settings: PermitHierarchicalResolution=ParametersOnly
  Feet Jacobians : Subsystem
  Mux : Mux  Inputs=2
  nu : Outport
  wires:
  w_H_b/1 -> Feet Jacobians/2(w_H_b)
  "feetInContact "/1 -> Compute Base Velocity/3(feetInContact)
  Mux/1 -> nu/1
  s/1 -> Feet Jacobians/1(s)
  Compute Base Velocity/1(nu_b) -> Mux/1
  sDot/1 -> Mux/2, Compute Base Velocity/4(sDot)
  Feet Jacobians/1(J_LFoot) -> Compute Base Velocity/1(J_LeftFoot)
  Feet Jacobians/2(J_RFoot) -> Compute Base Velocity/2(J_RightFoot)

== system torqueWalkingR2012b/Dynamics and Kinematics/Inverse Kinematics/ComputeTasksPoseAndVelocity ==
  J_LFoot : Inport
  J_RFoot : Inport  Port=2
  J_CoM : Inport  Port=3
  J_rot_task : Inport  Port=4
  J_LHand : Inport  Port=5
  J_RHand : Inport  Port=6
  qj : Inport  Port=7
  w_H_b : Inport  Port=8
  nu : Inport  Port=9
  Compose Task Pose and Velocity : MATLAB Function  TreatAsAtomicUnit=on
      settings: PermitHierarchicalResolution=ParametersOnly
  Product{,1..5} (6 alike) : Product  Multiplication=Matrix(*)
  Task position and orientation : Subsystem
  pose_vel_LFoot : Outport
  pose_vel_RFoot : Outport  Port=2
  pos_vel_CoM : Outport  Port=3
  orient_vel_rot_task : Outport  Port=4
  pose_vel_LHand : Outport  Port=5
  pose_vel_RHand : Outport  Port=6
  wires:
  Compose Task Pose and Velocity/2(pose_vel_RFoot) -> pose_vel_RFoot/1
  Compose Task Pose and Velocity/1(pose_vel_LFoot) -> pose_vel_LFoot/1
  Compose Task Pose and Velocity/3(pos_vel_CoM) -> pos_vel_CoM/1
  Compose Task Pose and Velocity/4(orient_vel_rot_task) -> orient_vel_rot_task/1
  nu/1 -> Product5/2, Product4/2, Product/2, Product1/2, Product2/2, Product3/2
  J_rot_task/1 -> Product3/1
  Product/1 -> Compose Task Pose and Velocity/3(vel_CoM)
  Product1/1 -> Compose Task Pose and Velocity/1(vel_LFoot)
  Product2/1 -> Compose Task Pose and Velocity/2(vel_RFoot)
  Product3/1 -> Compose Task Pose and Velocity/4(vel_rot_task)
  qj/1 -> Task position and orientation/1(s)
  w_H_b/1 -> Task position and orientation/2(w_H_b)
  Task position and orientation/3(w_H_CoM) -> Compose Task Pose and Velocity/9(w_H_CoM)
  Task position and orientation/1(w_H_l_sole) -> Compose Task Pose and Velocity/7(w_H_l_sole)
  Task position and orientation/2(w_H_r_sole) -> Compose Task Pose and Velocity/8(w_H_r_sole)
  Task position and orientation/4(w_H_rot_task) -> Compose Task Pose and Velocity/10(w_H_rot_task)
  J_LFoot/1 -> Product1/1
  J_CoM/1 -> Product/1
  J_RFoot/1 -> Product2/1
  J_LHand/1 -> Product4/1
  J_RHand/1 -> Product5/1
  Product4/1 -> Compose Task Pose and Velocity/5(vel_LHand)
  Product5/1 -> Compose Task Pose and Velocity/6(vel_RHand)
  Task position and orientation/5(w_H_l_hand) -> Compose Task Pose and Velocity/11(w_H_l_hand)
  Task position and orientation/6(w_H_r_hand) -> Compose Task Pose and Velocity/12(w_H_r_hand)
  Compose Task Pose and Velocity/5(pose_vel_LHand) -> pose_vel_LHand/1
  Compose Task Pose and Velocity/6(pose_vel_RHand) -> pose_vel_RHand/1

== system torqueWalkingR2012b/Dynamics and Kinematics/Inverse Kinematics/Jacobians and JDot_nu ==
  s : Inport
  w_H_b : Inport  Port=2
  nu_b : Inport  Port=3
  sDot : Inport  Port=4
  DotJ Nu CoM : WBToolboxLibrary/wholeBodyModel/Jacobians/DotJ Nu  frameName=Frames.COM  robotName=WBT_robotName  localName=WBT_modelName  wbiFile=WBT_wbiFilename  wbiList=WBT_wbiList
  DotJ Nu LFoot : WBToolboxLibrary/wholeBodyModel/Jacobians/DotJ Nu  frameName=Frames.LEFT_FOOT  robotName=WBT_robotName  localName=WBT_modelName  wbiFile=WBT_wbiFilename  wbiList=WBT_wbiList
  DotJ Nu LHand : WBToolboxLibrary/wholeBodyModel/Jacobians/DotJ Nu  frameName=Frames.LEFT_FOOT  robotName=WBT_robotName  localName=WBT_modelName  wbiFile=WBT_wbiFilename  wbiList=WBT_wbiList
  DotJ Nu RHand : WBToolboxLibrary/wholeBodyModel/Jacobians/DotJ Nu  frameName=Frames.RIGHT_FOOT  robotName=WBT_robotName  localName=WBT_modelName  wbiFile=WBT_wbiFilename  wbiList=WBT_wbiList
  DotJ Nu Rfoot : WBToolboxLibrary/wholeBodyModel/Jacobians/DotJ Nu  frameName=Frames.RIGHT_FOOT  robotName=WBT_robotName  localName=WBT_modelName  wbiFile=WBT_wbiFilename  wbiList=WBT_wbiList
  DotJ Nu rotational task : WBToolboxLibrary/wholeBodyModel/Jacobians/DotJ Nu  frameName=Frames.ROT_TASK_LINK  robotName=WBT_robotName  localName=WBT_modelName  wbiFile=WBT_wbiFilename  wbiList=WBT_wbiList
  Jacobian CoM : WBToolboxLibrary/wholeBodyModel/Jacobians/Jacobian  frameName=Frames.COM  robotName=WBT_robotName  localName=WBT_modelName  wbiFile=WBT_wbiFilename  wbiList=WBT_wbiList
  Jacobian LFoot : WBToolboxLibrary/wholeBodyModel/Jacobians/Jacobian  frameName=Frames.LEFT_FOOT  robotName=WBT_robotName  localName=WBT_modelName  wbiFile=WBT_wbiFilename  wbiList=WBT_wbiList
  Jacobian LFoot1 : WBToolboxLibrary/wholeBodyModel/Jacobians/Jacobian  frameName=Frames.LEFT_HAND  robotName=WBT_robotName  localName=WBT_modelName  wbiFile=WBT_wbiFilename  wbiList=WBT_wbiList
  Jacobian RFoot : WBToolboxLibrary/wholeBodyModel/Jacobians/Jacobian  frameName=Frames.RIGHT_FOOT  robotName=WBT_robotName  localName=WBT_modelName  wbiFile=WBT_wbiFilename  wbiList=WBT_wbiList
  Jacobian RFoot1 : WBToolboxLibrary/wholeBodyModel/Jacobians/Jacobian  frameName=Frames.RIGHT_HAND  robotName=WBT_robotName  localName=WBT_modelName  wbiFile=WBT_wbiFilename  wbiList=WBT_wbiList
  Jacobian rotational task : WBToolboxLibrary/wholeBodyModel/Jacobians/Jacobian  frameName=Frames.ROT_TASK_LINK  robotName=WBT_robotName  localName=WBT_modelName  wbiFile=WBT_wbiFilename  wbiList=WBT_wbiList
  J_LFoot : Outport
  J_RFoot : Outport  Port=2
  J_CoM : Outport  Port=3
  J_rot_task : Outport  Port=4
  J_LHand : Outport  Port=5
  J_RHand : Outport  Port=6
  JDot_nu_LFoot : Outport  Port=7
  JDot_nu_RFoot : Outport  Port=8
  JDot_nu_CoM : Outport  Port=9
  JDot_nu_rot_task : Outport  Port=10
  JDot_nu_LHand : Outport  Port=11
  JDot_nu_RHand : Outport  Port=12
  wires:
  Jacobian CoM/1 -> J_CoM/1
  Jacobian rotational task/1 -> J_rot_task/1
  Jacobian LFoot/1 -> J_LFoot/1
  Jacobian RFoot/1 -> J_RFoot/1
  w_H_b/1 -> Jacobian rotational task/1, Jacobian RFoot1/1, Jacobian LFoot1/1, Jacobian CoM/1, Jacobian RFoot/1, Jacobian LFoot/1, DotJ Nu CoM/1, DotJ Nu LHand/1, DotJ Nu RHand/1, DotJ Nu rotational task/1, DotJ Nu Rfoot/1, DotJ Nu LFoot/1
  sDot/1 -> DotJ Nu LFoot/4, DotJ Nu Rfoot/4, DotJ Nu RHand/4, DotJ Nu LHand/4, DotJ Nu rotational task/4, DotJ Nu CoM/4
  nu_b/1 -> DotJ Nu LHand/3, DotJ Nu RHand/3, DotJ Nu LFoot/3, DotJ Nu Rfoot/3, DotJ Nu CoM/3, DotJ Nu rotational task/3
  s/1 -> Jacobian rotational task/2, Jacobian RFoot1/2, Jacobian LFoot1/2, Jacobian CoM/2, Jacobian RFoot/2, Jacobian LFoot/2, DotJ Nu CoM/2, DotJ Nu LHand/2, DotJ Nu RHand/2, DotJ Nu rotational task/2, DotJ Nu Rfoot/2, DotJ Nu LFoot/2
  DotJ Nu Rfoot/1 -> JDot_nu_RFoot/1
  DotJ Nu LFoot/1 -> JDot_nu_LFoot/1
  DotJ Nu rotational task/1 -> JDot_nu_rot_task/1
  DotJ Nu CoM/1 -> JDot_nu_CoM/1
  Jacobian RFoot1/1 -> J_RHand/1
  Jacobian LFoot1/1 -> J_LHand/1
  DotJ Nu LHand/1 -> JDot_nu_LHand/1
  DotJ Nu RHand/1 -> JDot_nu_RHand/1

== system torqueWalkingR2012b/Dynamics and Kinematics/Inverse Kinematics/QP-Based Inverse Kinematics ==
  q_0 : Inport
  nu_0 : Inport  Port=2
  s_sDot_sDDot_ref : Inport  Port=3
  J : Inport  Port=4
  JDot_nu : Inport  Port=5
  acc_task_star : Inport  Port=6
  impedances : Inport  Port=7
  dampings : Inport  Port=8
  feetInContact : Inport  Port=9
  "Compute QP Hessian, gradient and constraints " : MATLAB Function  TreatAsAtomicUnit=on
      settings: PermitHierarchicalResolution=ParametersOnly
  DoFs converter1 : WBToolboxLibrary/Utilities/DoFs converter  yarp2WBIOption=From WBI to YARP  robotName=WBT_robotName  localName=WBT_modelName  wbiFile=WBT_wbiFilename  wbiList=WBT_wbiList
  QP Solver (inverse kinematics) : Subsystem
  QP output : Scope  NumInputPorts=6
      settings: TimeRange=14  ShowLegends=on  MaxDataPoints=5000  SaveToWorkspace=off  YMin=-0.16835~-0.01382~-0.00545~-0.54834~-0.44991~-1.00000  YMax=0.09227~0.00494~0.01312~0.27362~0.25517~1.00000  SampleTime=-1
  Selector1 : Selector  InputPortWidth=ROBOT_DOF+6  IndexOptions=Index vector (dialog)  Indices=[7:29]  OutputSizes=1
  Selector3 : Selector  InputPortWidth=ROBOT_DOF+16  IndexOptions=Index vector (dialog)  Indices=[17:ROBOT_DOF+16]  OutputSizes=1
  inverse kinematics integration : Subsystem
  s_sDot_sDDot_des : Outport
  ExitFlagQP : Outport  Port=2
  nuDot : Outport  Port=3
  q : Outport  Port=4
  nu : Outport  Port=5
  wires:
  q_0/1 -> inverse kinematics integration/3(q_0)
  nu_0/1 -> inverse kinematics integration/2(nu_0)
  QP Solver (inverse kinematics)/1(nuDot) -> Selector1/1, inverse kinematics integration/1(nuDot), nuDot/1
  "Compute QP Hessian, gradient and constraints "/4(biasVectorConstraint) -> QP Solver (inverse kinematics)/4(biasVectorConstraint)
  "Compute QP Hessian, gradient and constraints "/3(ConstraintMatrix) -> QP Solver (inverse kinematics)/3(ConstraintMatrix)
  "Compute QP Hessian, gradient and constraints "/2(gradient) -> QP Solver (inverse kinematics)/2(gradient)
  "Compute QP Hessian, gradient and constraints "/1(Hessian) -> QP Solver (inverse kinematics)/1(Hessian)
  impedances/1 -> "Compute QP Hessian, gradient and constraints "/4(impedances)
  dampings/1 -> "Compute QP Hessian, gradient and constraints "/5(dampings)
  s_sDot_sDDot_ref/1 -> "Compute QP Hessian, gradient and constraints "/3(s_sDot_sDDot_ref)
  inverse kinematics integration/3(s_sDot_sDDot_des) -> s_sDot_sDDot_des/1
  inverse kinematics integration/2(q) -> q/1, Selector3/1
  Selector3/1 -> "Compute QP Hessian, gradient and constraints "/1(s)
  QP Solver (inverse kinematics)/2(ExitFlagQP) -> QP output/6, ExitFlagQP/1
  inverse kinematics integration/1(nu) -> nu/1, "Compute QP Hessian, gradient and constraints "/2(nu)
  J/1 -> "Compute QP Hessian, gradient and constraints "/6(J)
  JDot_nu/1 -> "Compute QP Hessian, gradient and constraints "/7(JDot_nu)
  acc_task_star/1 -> "Compute QP Hessian, gradient and constraints "/8(acc_task_star)
  feetInContact/1 -> "Compute QP Hessian, gradient and constraints "/9(feetInContact)
  Selector1/1 -> DoFs converter1/1
  DoFs converter1/1 -> QP output/1
  DoFs converter1/2 -> QP output/2
  DoFs converter1/3 -> QP output/3
  DoFs converter1/4 -> QP output/4
  DoFs converter1/5 -> QP output/5
